simulink model "Paper_Threephase_Grid_PV"  (R2015a)
settings: Solver=ode23t  StartTime=0.0  StopTime=0.5  RelTol=1e-3
libraries: powerlib x32, powerlib_meascontrol x7, simulink x7, re_lib x1
settings Model: Creator=user  LastModifiedBy=user

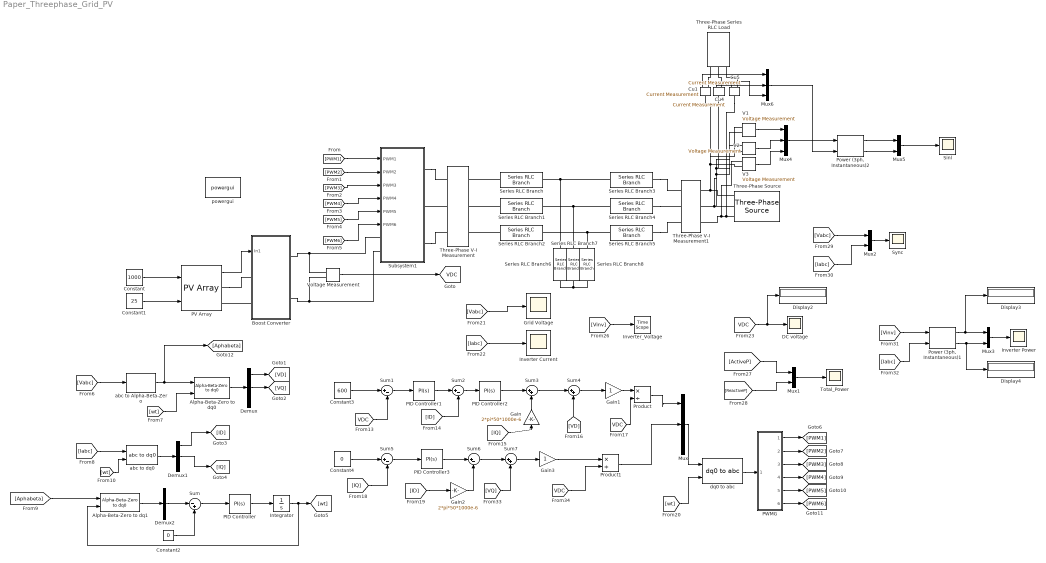
== system Paper_Threephase_Grid_PV ==
  Alpha-Beta-Zero to dq0 : powerlib_meascontrol/Transformations/Alpha-Beta-Zero to dq0  Alignment=90 degrees behind phase A axis
  Alpha-Beta-Zero to dq1 : powerlib_meascontrol/Transformations/Alpha-Beta-Zero to dq0  Alignment=90 degrees behind phase A axis
  Boost Converter : Subsystem
  Constant : Constant  Value=1000
  Constant1 : Constant  Value=25
  Constant2 : Constant  Value=0
  Constant3 : Constant  Value=600
  Constant4 : Constant  Value=0
  Cu1 : powerlib/Measurements/Current Measurement  PhasorSimulation=off  OutputType=Complex  PSBequivalent=0
  Cu4 : powerlib/Measurements/Current Measurement  PhasorSimulation=off  OutputType=Complex  PSBequivalent=0
  Cu5 : powerlib/Measurements/Current Measurement  PhasorSimulation=off  OutputType=Complex  PSBequivalent=0
  DC voltage : Scope
      settings: YMin=0  YMax=1300  SaveName=VDC
  Demux : Demux  Outputs=3
  Demux1 : Demux  Outputs=3
  Demux2 : Demux  Outputs=3
  Display2 : Display
  Display3 : Display
  Display4 : Display
  Gain : Gain  Gain=2*pi*50*1000e-6
  Gain1 : Gain
  Gain2 : Gain  Gain=2*pi*50*1000e-6
  Gain3 : Gain
  Grid Voltage : Scope
      settings: TickLabels=on  YMin=-600  YMax=600  SaveName=Grid
  Integrator : Integrator
  Inverter Current : Scope
      settings: TickLabels=on  YMin=-900  YMax=1100  SaveName=Grid1
  Inverter Power : Scope
      settings: TickLabels=on  YMin=-600000  YMax=700000  SaveName=Inverter_Power
  Inverter_Voltage : TimeScope
  Mux : Mux  Inputs=3
  Mux{1..3,5} (4 alike) : Mux  Inputs=2
  Mux4 : Mux  Inputs=3
  Mux6 : Mux  Inputs=3
  PID Controller : simulink/Continuous/PID Controller  Controller=PI  TimeDomain=Continuous-time  SampleTime=-1  IntegratorMethod=Forward Euler  FilterMethod=Forward Euler  Form=Parallel  UseFilter=on  ControllerParametersSource=internal  P=10  I=50000  D=0  N=100  InitialConditionSource=internal  InitialConditionForIntegrator=0  InitialConditionForFilter=0  ExternalReset=none  LimitOutput=off  UpperSaturationLimit=inf  LowerSaturationLimit=-inf  LinearizeAsGain=on  AntiWindupMode=none  Kb=1  TrackingMode=off  Kt=1  PParamMin=[]  PParamMax=[]  IParamMin=[]  IParamMax=[]  DParamMin=[]  DParamMax=[]  NParamMin=[]  NParamMax=[]  KbParamMin=[]  KbParamMax=[]  KtParamMin=[]  KtParamMax=[]  POutMin=[]  POutMax=[]  IOutMin=[]  IOutMax=[]  DOutMin=[]  DOutMax=[]  NOutMin=[]  NOutMax=[]  KbOutMin=[]  KbOutMax=[]  KtOutMin=[]  KtOutMax=[]  IntegratorOutMin=[]  IntegratorOutMax=[]  FilterOutMin=[]  FilterOutMax=[]  SumOutMin=[]  SumOutMax=[]  SumI1OutMin=[]  SumI1OutMax=[]  SumI2OutMin=[]  SumI2OutMax=[]  SumI3OutMin=[]  SumI3OutMax=[]  SumDOutMin=[]  SumDOutMax=[]  SaturationOutMin=[]  SaturationOutMax=[]  IntegratorContinuousStateAttributes=''  IntegratorStateMustResolveToSignalObject=off  IntegratorRTWStateStorageClass=Auto  FilterContinuousStateAttributes=''  FilterStateMustResolveToSignalObject=off  FilterRTWStateStorageClass=Auto  DifferentiatorICPrevScaledInput=0  DifferentiatorOutMin=[]  DifferentiatorOutMax=[]
  PID Controller1 : simulink/Continuous/PID Controller  Controller=PI  TimeDomain=Continuous-time  SampleTime=-1  IntegratorMethod=Forward Euler  FilterMethod=Forward Euler  Form=Parallel  UseFilter=on  ControllerParametersSource=internal  P=0.36  I=336  D=0  N=100  InitialConditionSource=internal  InitialConditionForIntegrator=0  InitialConditionForFilter=0  ExternalReset=none  LimitOutput=off  UpperSaturationLimit=inf  LowerSaturationLimit=-inf  LinearizeAsGain=on  AntiWindupMode=none  Kb=1  TrackingMode=off  Kt=1  PParamMin=[]  PParamMax=[]  IParamMin=[]  IParamMax=[]  DParamMin=[]  DParamMax=[]  NParamMin=[]  NParamMax=[]  KbParamMin=[]  KbParamMax=[]  KtParamMin=[]  KtParamMax=[]  POutMin=[]  POutMax=[]  IOutMin=[]  IOutMax=[]  DOutMin=[]  DOutMax=[]  NOutMin=[]  NOutMax=[]  KbOutMin=[]  KbOutMax=[]  KtOutMin=[]  KtOutMax=[]  IntegratorOutMin=[]  IntegratorOutMax=[]  FilterOutMin=[]  FilterOutMax=[]  SumOutMin=[]  SumOutMax=[]  SumI1OutMin=[]  SumI1OutMax=[]  SumI2OutMin=[]  SumI2OutMax=[]  SumI3OutMin=[]  SumI3OutMax=[]  SumDOutMin=[]  SumDOutMax=[]  SaturationOutMin=[]  SaturationOutMax=[]  IntegratorContinuousStateAttributes=''  IntegratorStateMustResolveToSignalObject=off  IntegratorRTWStateStorageClass=Auto  FilterContinuousStateAttributes=''  FilterStateMustResolveToSignalObject=off  FilterRTWStateStorageClass=Auto  DifferentiatorICPrevScaledInput=0  DifferentiatorOutMin=[]  DifferentiatorOutMax=[]
  PID Controller2 : simulink/Continuous/PID Controller  Controller=PI  TimeDomain=Continuous-time  SampleTime=-1  IntegratorMethod=Forward Euler  FilterMethod=Forward Euler  Form=Parallel  UseFilter=on  ControllerParametersSource=internal  P=10  I=20  D=0  N=100  InitialConditionSource=internal  InitialConditionForIntegrator=0  InitialConditionForFilter=0  ExternalReset=none  LimitOutput=off  UpperSaturationLimit=inf  LowerSaturationLimit=-inf  LinearizeAsGain=on  AntiWindupMode=none  Kb=1  TrackingMode=off  Kt=1  PParamMin=[]  PParamMax=[]  IParamMin=[]  IParamMax=[]  DParamMin=[]  DParamMax=[]  NParamMin=[]  NParamMax=[]  KbParamMin=[]  KbParamMax=[]  KtParamMin=[]  KtParamMax=[]  POutMin=[]  POutMax=[]  IOutMin=[]  IOutMax=[]  DOutMin=[]  DOutMax=[]  NOutMin=[]  NOutMax=[]  KbOutMin=[]  KbOutMax=[]  KtOutMin=[]  KtOutMax=[]  IntegratorOutMin=[]  IntegratorOutMax=[]  FilterOutMin=[]  FilterOutMax=[]  SumOutMin=[]  SumOutMax=[]  SumI1OutMin=[]  SumI1OutMax=[]  SumI2OutMin=[]  SumI2OutMax=[]  SumI3OutMin=[]  SumI3OutMax=[]  SumDOutMin=[]  SumDOutMax=[]  SaturationOutMin=[]  SaturationOutMax=[]  IntegratorContinuousStateAttributes=''  IntegratorStateMustResolveToSignalObject=off  IntegratorRTWStateStorageClass=Auto  FilterContinuousStateAttributes=''  FilterStateMustResolveToSignalObject=off  FilterRTWStateStorageClass=Auto  DifferentiatorICPrevScaledInput=0  DifferentiatorOutMin=[]  DifferentiatorOutMax=[]
  PID Controller3 : simulink/Continuous/PID Controller  Controller=PI  TimeDomain=Continuous-time  SampleTime=-1  IntegratorMethod=Forward Euler  FilterMethod=Forward Euler  Form=Parallel  UseFilter=on  ControllerParametersSource=internal  P=10  I=20  D=0  N=100  InitialConditionSource=internal  InitialConditionForIntegrator=0  InitialConditionForFilter=0  ExternalReset=none  LimitOutput=off  UpperSaturationLimit=inf  LowerSaturationLimit=-inf  LinearizeAsGain=on  AntiWindupMode=none  Kb=1  TrackingMode=off  Kt=1  PParamMin=[]  PParamMax=[]  IParamMin=[]  IParamMax=[]  DParamMin=[]  DParamMax=[]  NParamMin=[]  NParamMax=[]  KbParamMin=[]  KbParamMax=[]  KtParamMin=[]  KtParamMax=[]  POutMin=[]  POutMax=[]  IOutMin=[]  IOutMax=[]  DOutMin=[]  DOutMax=[]  NOutMin=[]  NOutMax=[]  KbOutMin=[]  KbOutMax=[]  KtOutMin=[]  KtOutMax=[]  IntegratorOutMin=[]  IntegratorOutMax=[]  FilterOutMin=[]  FilterOutMax=[]  SumOutMin=[]  SumOutMax=[]  SumI1OutMin=[]  SumI1OutMax=[]  SumI2OutMin=[]  SumI2OutMax=[]  SumI3OutMin=[]  SumI3OutMax=[]  SumDOutMin=[]  SumDOutMax=[]  SaturationOutMin=[]  SaturationOutMax=[]  IntegratorContinuousStateAttributes=''  IntegratorStateMustResolveToSignalObject=off  IntegratorRTWStateStorageClass=Auto  FilterContinuousStateAttributes=''  FilterStateMustResolveToSignalObject=off  FilterRTWStateStorageClass=Auto  DifferentiatorICPrevScaledInput=0  DifferentiatorOutMin=[]  DifferentiatorOutMax=[]
  PV Array : re_lib/Solar/PV Array  Npar=47  Nser=10  PlotType=array @ 25 deg.C & specified irradiances  S_vec="[ 1000  800 500  100 ]"  Temp_C_vec="[ 45 25  ]"  ModuleName=1Soltech 1STH-215-P  PlotWhenSelected=off  Pm=213.15  Ncell=60  Voc=36.3  Isc=7.84  Vm=29  Im=7.35  beta_Voc_pc=-0.36099  alpha_Isc_pc=0.102  beta_Voc=-0.13104  alpha_Isc=0.007997  IL=7.8649  I0=2.9259e-10  nI=0.98117  Rsh=313.3991  Rs=0.39383  BAL=on  Tc=1e-6  Tfilter=1e-6
  PWMG : Subsystem
  "Power (3ph, Instantaneous)1" : powerlib_meascontrol/Measurements/Power (3ph, Instantaneous)
  "Power (3ph, Instantaneous)2" : powerlib_meascontrol/Measurements/Power (3ph, Instantaneous)
  Product : Product  Inputs=*/
  Product1 : Product  Inputs=*/
  Series RLC Branch{,1..5} (6 alike) : powerlib/Elements/Series RLC Branch  LConnTagsString=__new0  RConnTagsString=__new0  BranchType=RL  Resistance=1e-3  Inductance=500e-6  SetiL0=off  InitialCurrent=0  Capacitance=1e-6  Setx0=off  InitialVoltage=0  Measurements=None
  Series RLC Branch6 : powerlib/Elements/Series RLC Branch  LConnTagsString=__new0  RConnTagsString=__new0  BranchType=RC  Resistance=1e-3  Inductance=500e-6  SetiL0=off  InitialCurrent=0  Capacitance=100e-6  Setx0=off  InitialVoltage=0  Measurements=None
  Series RLC Branch7 : powerlib/Elements/Series RLC Branch  LConnTagsString=__new0  RConnTagsString=__new0  BranchType=RC  Resistance=1e-3  Inductance=500e-6  SetiL0=off  InitialCurrent=0  Capacitance=100e-6  Setx0=off  InitialVoltage=0  Measurements=None
  Series RLC Branch8 : powerlib/Elements/Series RLC Branch  LConnTagsString=__new0  RConnTagsString=__new0  BranchType=RC  Resistance=1e-3  Inductance=500e-6  SetiL0=off  InitialCurrent=0  Capacitance=100e-6  Setx0=off  InitialVoltage=0  Measurements=None
  Sinl : Scope
      settings: YMin=-10000  YMax=140000  SaveName=Sink
  Subsystem1 : Subsystem
  Sum : Sum  Inputs=|-+
  Sum{1..2,5..6} (4 alike) : Sum  Inputs=|+-
  Sum3 : Sum  Inputs=|++
  Sum4 : Sum  Inputs=|++
  Sum7 : Sum  Inputs=|++
  Sync : Scope
      settings: YMin=-800  YMax=800  SaveName=TotalPV_Power1
  Three-Phase Series RLC Load : powerlib/Elements/Three-Phase Series RLC Load  LConnTagsString=A|B|C  Configuration=Y (grounded)  NominalVoltage=400  NominalFrequency=50  ActivePower=10e3  InductivePower=8e3  CapacitivePower=0  Measurements=None  LoadType=constant Z
  Three-Phase V-I Measurement : powerlib/Measurements/Three-Phase V-I Measurement  VoltageMeasurement=phase-to-ground  SetLabelV=on  LabelV=Vinv  Vpu=off  VpuLL=off  CurrentMeasurement=yes  SetLabelI=on  LabelI=Iabc  Ipu=off  Pbase=100e6  Vbase=500e3  OutputType=Complex  PhasorSimulation=off  PSBequivalent=0
  Three-Phase V-I Measurement1 : powerlib/Measurements/Three-Phase V-I Measurement  VoltageMeasurement=phase-to-ground  SetLabelV=on  LabelV=Vabc  Vpu=off  VpuLL=off  CurrentMeasurement=yes  SetLabelI=on  LabelI=Igrid  Ipu=off  Pbase=100e6  Vbase=500e3  OutputType=Complex  PhasorSimulation=off  PSBequivalent=0
  Three-Phase Source : powerlib/Electrical Sources/Three-Phase Source  Voltage=400  PhaseAngle=0  Frequency=50  InternalConnection=Yg  SpecifyImpedance=off  Resistance=1e-6  Inductance=1e-6  ShortCircuitLevel=100e6  BaseVoltage=400  XRratio=7  BusType=swing  Pref=0  Qref=0  Qmin=-inf  Qmax=inf
  Total_Power : Scope
      settings: YMin=-500000  YMax=350000  SaveName=TotalPV_Power
  V1 : powerlib/Measurements/Voltage Measurement  PhasorSimulation=off  OutputType=Complex  PSBequivalent=0
  V2 : powerlib/Measurements/Voltage Measurement  PhasorSimulation=off  OutputType=Complex  PSBequivalent=0
  V3 : powerlib/Measurements/Voltage Measurement  PhasorSimulation=off  OutputType=Complex  PSBequivalent=0
  Voltage Measurement : powerlib/Measurements/Voltage Measurement  PhasorSimulation=off  OutputType=Complex  PSBequivalent=0
  abc to Alpha-Beta-Zero : powerlib_meascontrol/Transformations/abc to Alpha-Beta-Zero
  abc to dq0 : powerlib_meascontrol/Transformations/abc to dq0  Alignment=90 degrees behind phase A axis
  dq0 to abc : powerlib_meascontrol/Transformations/dq0 to abc  Alignment=90 degrees behind phase A axis
  powergui : powerlib/powergui  Priority=1  SimulationMode=Discrete  SolverType=Tustin/Backward Euler (TBE)  SampleTime=1e-6  frequency=60  SPID=off  DisableSnubberDevices=off  DisableRonSwitches=off  DisableVfSwitches=off  SwTol=0  DisplayEquations=off  Interpol=off  methode=off  Ts=100  FunctionMessages=off  echomessages=off  HookPort=off  EnableUseOfTLC=off  x0status=blocks  frequencyindice=50  Pbase=100e6  ErrMax=1e-4  Iterations=50  UnitsV=kV  UnitsW=MW  buscounter=0  RestoreLinks=warning  ResistiveCurrentMeasurement=off  Frange=[0:2:500]  Ylog=off  Xlog=on  ShowGrid=off  save=off  variable=ZData  structure=Grid  ZoomFFT=off  StartTime=0.0  cycles=10  DisplayStyle=1  fundamental=50  FreqAxis=on  MaxFrequency=1000  frequencyindicesteady=1  RmsSteady=1  display=off
  tag scope: VDC=global
  wires:
  Constant/1 -> PV Array/1
  Constant1/1 -> PV Array/2
  PV Array/1 -> Boost Converter/1(In1)
  [PWM1] -> Subsystem1/1(PWM1)
  [PWM2] -> Subsystem1/2(PWM2)
  [PWM3] -> Subsystem1/3(PWM3)
  [PWM4] -> Subsystem1/4(PWM4)
  [PWM5] -> Subsystem1/5(PWM5)
  [PWM6] -> Subsystem1/6(PWM6)
  Voltage Measurement/1 -> [VDC]
  [wt] -> Alpha-Beta-Zero to dq0/2
  Alpha-Beta-Zero to dq0/1 -> Demux/1
  Demux/2 -> [VQ]
  Demux/1 -> [VD]
  [Iabc] -> abc to dq0/1
  abc to dq0/1 -> Demux1/1
  Demux1/1 -> [ID]
  Demux1/2 -> [IQ]
  [wt] -> abc to dq0/2
  Alpha-Beta-Zero to dq1/1 -> Demux2/1
  Demux2/2 -> Sum/1
  Constant2/1 -> Sum/2
  Sum/1 -> PID Controller/1
  PID Controller/1 -> Integrator/1
  Integrator/1 -> [wt], Alpha-Beta-Zero to dq1/2
  PWMG/1(PWM1) -> [PWM1]
  PWMG/2(PWM2) -> [PWM2]
  PWMG/3(PWM3) -> [PWM3]
  PWMG/4(PWM4) -> [PWM4]
  PWMG/5(PWM5) -> [PWM5]
  PWMG/6(PWM6) -> [PWM6]
  [VDC] -> Display2/1, DC voltage/1
  dq0 to abc/1 -> PWMG/1(Vref)
  [wt] -> dq0 to abc/2
  [Vabc] -> abc to Alpha-Beta-Zero/1
  abc to Alpha-Beta-Zero/1 -> [Aphabeta], Alpha-Beta-Zero to dq0/1
  [Aphabeta] -> Alpha-Beta-Zero to dq1/1
  [Vinv] -> Inverter_Voltage/1
  [Vabc] -> Grid Voltage/1
  [Iabc] -> Inverter Current/1
  [ActiveP] -> Mux1/1
  Mux1/1 -> Total_Power/1
  [ReactiveP] -> Mux1/2
  Mux2/1 -> Sync/1
  [Vabc] -> Mux2/1
  [Iabc] -> Mux2/2
  [Vinv] -> "Power (3ph, Instantaneous)1"/1
  [Iabc] -> "Power (3ph, Instantaneous)1"/2
  "Power (3ph, Instantaneous)1"/1 -> Display3/1, Mux3/1
  "Power (3ph, Instantaneous)1"/2 -> Display4/1, Mux3/2
  Mux3/1 -> Inverter Power/1
  [ID] -> Sum2/2
  [VDC] -> Sum1/2
  Constant3/1 -> Sum1/1
  Sum1/1 -> PID Controller1/1
  PID Controller2/1 -> Sum3/1
  PID Controller1/1 -> Sum2/1
  Sum2/1 -> PID Controller2/1
  Sum3/1 -> Sum4/1
  [VD] -> Sum4/2
  Gain/1 -> Sum3/2
  Gain2/1 -> Sum6/2
  Gain3/1 -> Product1/1
  Sum7/1 -> Gain3/1
  [VDC] -> Product1/2
  Constant4/1 -> Sum5/1
  [VDC] -> Product/2
  Sum5/1 -> PID Controller3/1
  PID Controller3/1 -> Sum6/1
  [ID] -> Gain2/1
  Sum6/1 -> Sum7/1
  [IQ] -> Gain/1
  Gain1/1 -> Product/1
  Sum4/1 -> Gain1/1
  [IQ] -> Sum5/2
  [VQ] -> Sum7/2
  Product/1 -> Mux/1
  Product1/1 -> Mux/2
  Mux/1 -> dq0 to abc/1
  V1/1 -> Mux4/1
  V2/1 -> Mux4/2
  V3/1 -> Mux4/3
  Mux4/1 -> "Power (3ph, Instantaneous)2"/1
  Mux5/1 -> Sinl/1
  "Power (3ph, Instantaneous)2"/1 -> Mux5/1
  Cu1/1 -> Mux6/1
  Cu4/1 -> Mux6/2
  Cu5/1 -> Mux6/3
  Mux6/1 -> "Power (3ph, Instantaneous)2"/2
  "Power (3ph, Instantaneous)2"/2 -> Mux5/2
  connections:
  Boost Converter/LConn2 -- PV Array/RConn2
  PV Array/RConn1 -- Boost Converter/LConn1
  Voltage Measurement/LConn2 -- Subsystem1/LConn2 -- Boost Converter/RConn2
  Boost Converter/RConn1 -- Subsystem1/LConn1 -- Voltage Measurement/LConn1
  Three-Phase V-I Measurement/LConn2 -- Subsystem1/RConn2
  Subsystem1/RConn1 -- Three-Phase V-I Measurement/LConn1
  Subsystem1/RConn3 -- Three-Phase V-I Measurement/LConn3
  Series RLC Branch/LConn1 -- Three-Phase V-I Measurement/RConn1
  Series RLC Branch1/LConn1 -- Three-Phase V-I Measurement/RConn2
  Series RLC Branch2/LConn1 -- Three-Phase V-I Measurement/RConn3
  Series RLC Branch3/LConn1 -- Series RLC Branch6/LConn1 -- Series RLC Branch/RConn1
  Series RLC Branch4/LConn1 -- Series RLC Branch7/LConn1 -- Series RLC Branch1/RConn1
  Series RLC Branch5/LConn1 -- Series RLC Branch8/LConn1 -- Series RLC Branch2/RConn1
  Series RLC Branch6/RConn1 -- Series RLC Branch7/RConn1 -- Series RLC Branch8/RConn1
  Series RLC Branch4/RConn1 -- Three-Phase V-I Measurement1/RConn2
  Series RLC Branch3/RConn1 -- Three-Phase V-I Measurement1/RConn1
  Series RLC Branch5/RConn1 -- Three-Phase V-I Measurement1/RConn3
  Three-Phase Source/RConn3 -- V1/LConn1 -- Cu1/LConn1 -- V3/LConn2 -- Three-Phase V-I Measurement1/LConn1
  Three-Phase Source/RConn2 -- Cu4/LConn1 -- V1/LConn2 -- V2/LConn1 -- V2/LConn2 -- Three-Phase V-I Measurement1/LConn2
  Three-Phase Source/RConn1 -- V3/LConn1 -- Three-Phase V-I Measurement1/LConn3 -- Cu5/LConn1
  Cu1/RConn1 -- Three-Phase Series RLC Load/LConn1
  Cu4/RConn1 -- Three-Phase Series RLC Load/LConn2
  Cu5/RConn1 -- Three-Phase Series RLC Load/LConn3

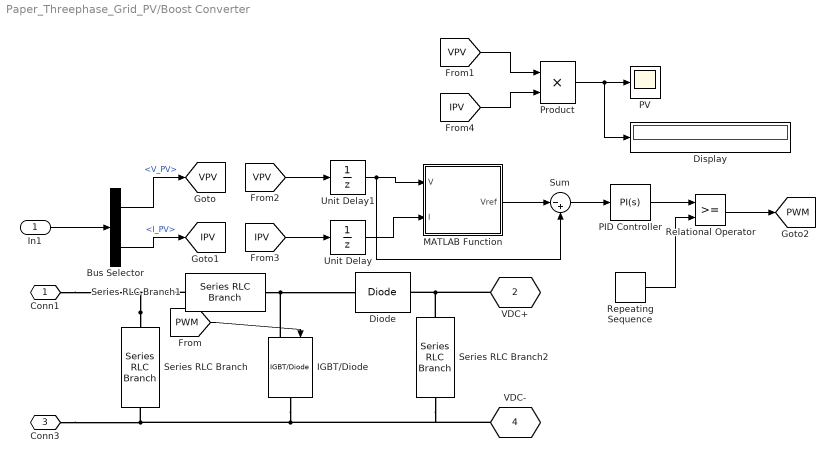
== system Paper_Threephase_Grid_PV/Boost Converter ==
  In1 : Inport
  Bus Selector : BusSelector  OutputSignals=V_PV,I_PV
  Diode : powerlib/Power Electronics/Diode  Ron=0.001  Lon=0  Vf=0.8  IC=0  UseSnubber=off  Rs=500  Cs=250e-9  Measurements=off
  Display : Display
  IGBT/Diode : powerlib/Power Electronics/IGBT//Diode  Ron=1e-3  Rs=1e5  Cs=inf  Measurements=off
  MATLAB Function : MATLAB Function  TreatAsAtomicUnit=on
  PID Controller : simulink/Continuous/PID Controller  Controller=PI  TimeDomain=Continuous-time  SampleTime=-1  IntegratorMethod=Forward Euler  FilterMethod=Forward Euler  Form=Parallel  UseFilter=on  ControllerParametersSource=internal  P=0.005  I=0.001  D=0  N=100  InitialConditionSource=internal  InitialConditionForIntegrator=0  InitialConditionForFilter=0  ExternalReset=none  LimitOutput=on  UpperSaturationLimit=0.95  LowerSaturationLimit=0  LinearizeAsGain=on  AntiWindupMode=none  Kb=1  TrackingMode=off  Kt=1  PParamMin=[]  PParamMax=[]  IParamMin=[]  IParamMax=[]  DParamMin=[]  DParamMax=[]  NParamMin=[]  NParamMax=[]  KbParamMin=[]  KbParamMax=[]  KtParamMin=[]  KtParamMax=[]  POutMin=[]  POutMax=[]  IOutMin=[]  IOutMax=[]  DOutMin=[]  DOutMax=[]  NOutMin=[]  NOutMax=[]  KbOutMin=[]  KbOutMax=[]  KtOutMin=[]  KtOutMax=[]  IntegratorOutMin=[]  IntegratorOutMax=[]  FilterOutMin=[]  FilterOutMax=[]  SumOutMin=[]  SumOutMax=[]  SumI1OutMin=[]  SumI1OutMax=[]  SumI2OutMin=[]  SumI2OutMax=[]  SumI3OutMin=[]  SumI3OutMax=[]  SumDOutMin=[]  SumDOutMax=[]  SaturationOutMin=[]  SaturationOutMax=[]  IntegratorContinuousStateAttributes=''  IntegratorStateMustResolveToSignalObject=off  IntegratorRTWStateStorageClass=Auto  FilterContinuousStateAttributes=''  FilterStateMustResolveToSignalObject=off  FilterRTWStateStorageClass=Auto  DifferentiatorICPrevScaledInput=0  DifferentiatorOutMin=[]  DifferentiatorOutMax=[]
  PV : Scope
      settings: YMin=-125000  YMax=125000  SaveName=MPPT
  Product : Product
  Relational Operator : RelationalOperator  OutDataTypeStr=boolean
  Repeating Sequence : simulink/Sources/Repeating Sequence  rep_seq_t=[0 0.0002]  rep_seq_y=[0 1]
  Series RLC Branch : powerlib/Elements/Series RLC Branch  LConnTagsString=__new0  RConnTagsString=__new0  BranchType=RC  Resistance=1e-3  Inductance=1e-3  SetiL0=off  InitialCurrent=0  Capacitance=1000e-6  Setx0=off  InitialVoltage=0  Measurements=None
  Series RLC Branch1 : powerlib/Elements/Series RLC Branch  LConnTagsString=__new0  RConnTagsString=__new0  BranchType=L  Resistance=1e-3  Inductance=1.45e-3  SetiL0=off  InitialCurrent=0  Capacitance=1000e-6  Setx0=off  InitialVoltage=0  Measurements=None
  Series RLC Branch2 : powerlib/Elements/Series RLC Branch  LConnTagsString=__new0  RConnTagsString=__new0  BranchType=C  Resistance=1e-3  Inductance=1e-3  SetiL0=off  InitialCurrent=0  Capacitance=3227e-6  Setx0=off  InitialVoltage=0  Measurements=None
  Sum : Sum  Inputs=|-+
  Unit Delay : UnitDelay  SampleTime=1e-6
  Unit Delay1 : UnitDelay  SampleTime=1e-6
  Conn1 : PMIOPort  Port=1  Side=Left
  VDC+ : PMIOPort  Port=2  Side=Right
  Conn3 : PMIOPort  Port=3  Side=Left
  VDC- : PMIOPort  Port=4  Side=Right
  tag scope: IPV=global, PWM=global, VPV=global
  wires:
  In1/1 -> Bus Selector/1
  Bus Selector/2 -> [IPV]  "<I_PV>"
  [PWM] -> IGBT/Diode/1
  Unit Delay1/1 -> Sum/2, MATLAB Function/1(V)
  [VPV] -> Unit Delay1/1
  MATLAB Function/1(Vref) -> Sum/1
  Bus Selector/1 -> [VPV]  "<V_PV>"
  PID Controller/1 -> Relational Operator/1
  Repeating Sequence/1 -> Relational Operator/2
  Relational Operator/1 -> [PWM]
  Unit Delay/1 -> MATLAB Function/2(I)
  Sum/1 -> PID Controller/1
  [IPV] -> Unit Delay/1
  [VPV] -> Product/1
  [IPV] -> Product/2
  Product/1 -> Display/1, PV/1
  connections:
  Series RLC Branch1/RConn1 -- IGBT/Diode/LConn1 -- Diode/LConn1
  Series RLC Branch/RConn1 -- VDC-/RConn1 -- Series RLC Branch2/RConn1 -- IGBT/Diode/RConn1 -- Conn3/RConn1
  Series RLC Branch/LConn1 -- Conn1/RConn1 -- Series RLC Branch1/LConn1
  Series RLC Branch2/LConn1 -- VDC+/RConn1 -- Diode/RConn1

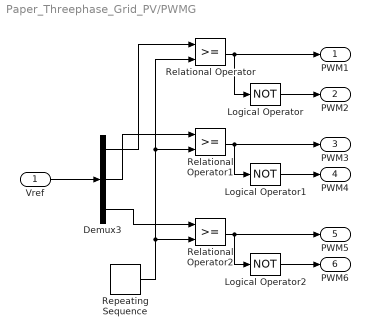
== system Paper_Threephase_Grid_PV/PWMG ==
  Vref : Inport
  Demux3 : Demux  Outputs=3
  Logical Operator : Logic  Operator=NOT  AllPortsSameDT=off  OutDataTypeStr=boolean
  Logical Operator1 : Logic  Operator=NOT  AllPortsSameDT=off  OutDataTypeStr=boolean
  Logical Operator2 : Logic  Operator=NOT  AllPortsSameDT=off  OutDataTypeStr=boolean
  Relational Operator : RelationalOperator  OutDataTypeStr=boolean
  Relational Operator1 : RelationalOperator  OutDataTypeStr=boolean
  Relational Operator2 : RelationalOperator  OutDataTypeStr=boolean
  Repeating Sequence : simulink/Sources/Repeating Sequence  rep_seq_t=[0 0.00005 0.0001]  rep_seq_y=[-1 1 -1]
  PWM1 : Outport
  PWM2 : Outport  Port=2
  PWM3 : Outport  Port=3
  PWM4 : Outport  Port=4
  PWM5 : Outport  Port=5
  PWM6 : Outport  Port=6
  wires:
  Relational Operator/1 -> PWM1/1, Logical Operator/1
  Demux3/2 -> Relational Operator1/1
  Logical Operator/1 -> PWM2/1
  Logical Operator1/1 -> PWM4/1
  Demux3/3 -> Relational Operator2/1
  Relational Operator2/1 -> PWM5/1, Logical Operator2/1
  Relational Operator1/1 -> PWM3/1, Logical Operator1/1
  Logical Operator2/1 -> PWM6/1
  Vref/1 -> Demux3/1
  Demux3/1 -> Relational Operator/1
  Repeating Sequence/1 -> Relational Operator2/2, Relational Operator1/2, Relational Operator/2

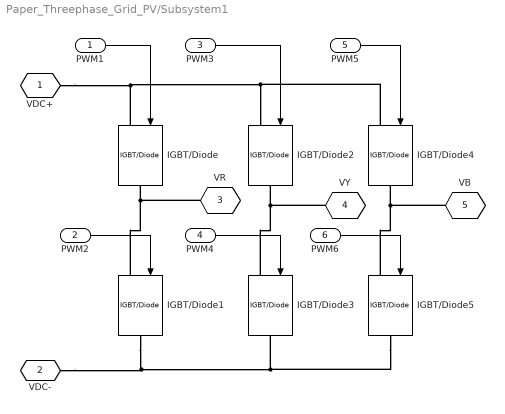
== system Paper_Threephase_Grid_PV/Subsystem1 ==
  PWM1 : Inport
  PWM2 : Inport  Port=2
  PWM3 : Inport  Port=3
  PWM4 : Inport  Port=4
  PWM5 : Inport  Port=5
  PWM6 : Inport  Port=6
  IGBT/Diode{,1..5} (6 alike) : powerlib/Power Electronics/IGBT//Diode  Ron=1e-3  Rs=1e5  Cs=inf  Measurements=off
  VDC+ : PMIOPort  Tag=PMCPort  Port=1  Side=Left
  VDC- : PMIOPort  Tag=PMCPort  Port=2  Side=Left
  VR : PMIOPort  Port=3  Side=Right
  VY : PMIOPort  Port=4  Side=Right
  VB : PMIOPort  Port=5  Side=Right
  wires:
  PWM4/1 -> IGBT/Diode3/1
  PWM2/1 -> IGBT/Diode1/1
  PWM3/1 -> IGBT/Diode2/1
  PWM5/1 -> IGBT/Diode4/1
  PWM6/1 -> IGBT/Diode5/1
  PWM1/1 -> IGBT/Diode/1
  connections:
  IGBT/Diode1/LConn1 -- VR/RConn1 -- IGBT/Diode/RConn1
  IGBT/Diode/LConn1 -- VDC+/RConn1 -- IGBT/Diode4/LConn1 -- IGBT/Diode2/LConn1
  IGBT/Diode1/RConn1 -- VDC-/RConn1 -- IGBT/Diode5/RConn1 -- IGBT/Diode3/RConn1
  IGBT/Diode3/LConn1 -- VY/RConn1 -- IGBT/Diode2/RConn1
  IGBT/Diode5/LConn1 -- VB/RConn1 -- IGBT/Diode4/RConn1

== matlab function Paper_Threephase_Grid_PV/Boost Converter/MATLAB Function ==
  data: V input; Vref output; I input
function Vref = RefGen(V,I)

Vrefmax=363;
Vrefmin=0.0;
Vrefini=300;
deltaVref=5;
persistent Vold Pold Vrefold;

dataType='double';

if isempty(Vold)
    Vold=0;
    Pold=0;
    Vrefold=Vrefini;
end
P=V*I;
dV=V-Vold;
dP=P-Pold;

if dP~=0
    if dP<0
        if dV<0
            Vref=Vrefold+deltaVref;
        else
            Vref=Vrefold-deltaVref;
        end
    else
        if dV<0
            Vref=Vrefold-deltaVref;
        else
            Vref=Vrefold+deltaVref;
        end
    end
else
    Vref=Vrefold;
end
if Vref>=Vrefmax | Vref<= Vrefmin
    Vref=Vrefold;
end
Vrefold=Vref;
Vold= V;
Pold=P;
